simulink model "BCIBLOCK"  (R2022b)
settings: Solver=VariableStepAuto  StartTime=0.0  StopTime=10.0  RelTol=1e-3
settings Model: Creator=music  LastModifiedBy=music

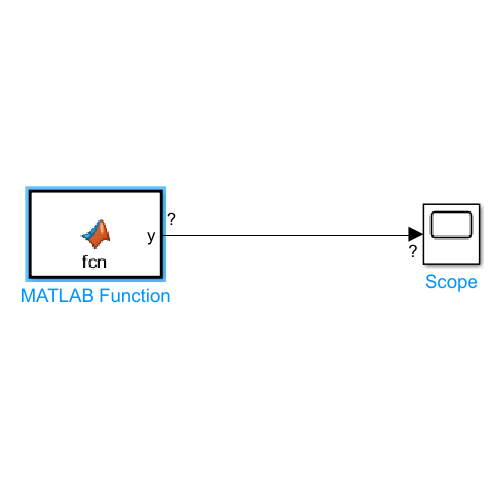
[thumbnail: Simulink's stored preview of the top-level diagram]
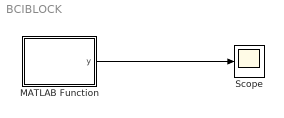
== system BCIBLOCK ==
  MATLAB Function : MATLAB Function  TreatAsAtomicUnit=on
  Scope : Scope
  wires:
  MATLAB Function/1(y) -> Scope/1

== matlab function BCIBLOCK/MATLAB Function ==
  data: y output
function y = fcn()

y= bci_connect();

end
